simulink model "Six_DoF_LQR"  (R2020b)
settings: Solver=VariableStepAuto  StartTime=0.0  StopTime=6  RelTol=1e-3
values from neighbouring files (symbols this model uses):
  D = zeros(3,2)    [ss_3DoF_LQR.m]    (also in ss_6DoF_LQR.m = zeros(6,2))
  inertiaxx = 0.0015    [Data_for_simulation.m]
  inertiayy = 0.048    [Data_for_simulation.m]
  inertiazz = 0.048    [Data_for_simulation.m]
  K = lqr(A,B,Q,R)    [ss_3DoF_LQR.m]    (also in ss_6DoF_LQR.m)
  mass = 0.8426    [Data_for_simulation.m]
  moment_arm = 0.29    [Data_for_simulation.m]
  tvc_misang = 0    [Data_for_simulation.m]
libraries: simulink_extras x3, shared6dof x1, aerolibutil x1, sharedutil x1
settings Model: Creator=tushark  LastModifiedBy=tushark

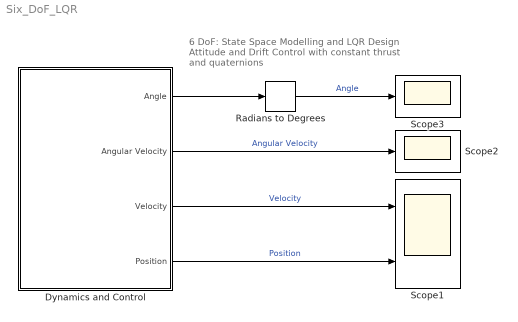
== system Six_DoF_LQR ==
  note: 6 DoF: State Space Modelling and LQR Design
      | Attitude and Drift Control with constant thrust and quaternions
  Dynamics and Control : Subsystem
  Radians to Degrees : simulink_extras/Transformations/Radians to Degrees
  Scope1 : Scope  NumInputPorts=2
  Scope2 : Scope
  Scope3 : Scope
  wires:
  Dynamics and Control/1(Angle) -> Radians to Degrees/1
  Dynamics and Control/2(Angular Velocity) -> Scope2/1  "Angular Velocity"
  Dynamics and Control/3(Velocity) -> Scope1/1  "Velocity"
  Radians to Degrees/1 -> Scope3/1  "Angle"
  Dynamics and Control/4(Position) -> Scope1/2  "Position"

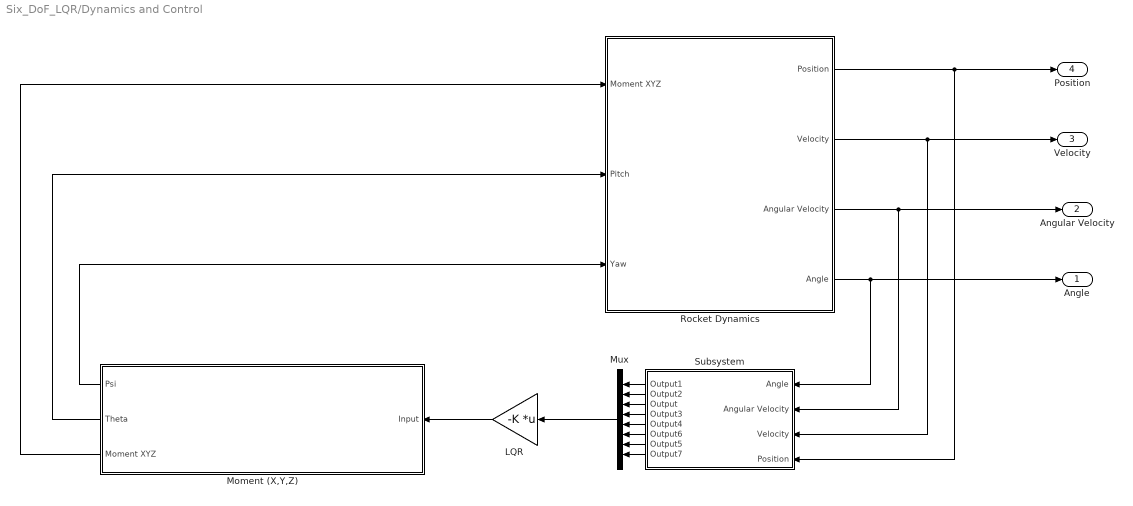
== system Six_DoF_LQR/Dynamics and Control ==
  LQR : Gain  Gain=-K  Multiplication=Matrix(K*u)
  Moment (X,Y,Z) : Subsystem
  Mux : Mux  Inputs=8
  Rocket Dynamics : Subsystem
  Subsystem : Subsystem
  Angle : Outport
  Angular Velocity : Outport  Port=2
  Velocity : Outport  Port=3
  Position : Outport  Port=4
  wires:
  Rocket Dynamics/3(Angular Velocity) -> Angular Velocity/1, Subsystem/2(Angular Velocity)
  Rocket Dynamics/2(Velocity) -> Subsystem/3(Velocity), Velocity/1
  Mux/1 -> LQR/1
  LQR/1 -> Moment (X,Y,Z)/1("Input ")
  Moment (X,Y,Z)/1(Psi) -> Rocket Dynamics/3(Yaw)
  Moment (X,Y,Z)/2(Theta) -> Rocket Dynamics/2(Pitch)
  Moment (X,Y,Z)/3(Moment XYZ) -> Rocket Dynamics/1(Moment XYZ)
  Rocket Dynamics/1(Position) -> Subsystem/4(Position), Position/1
  Rocket Dynamics/4(Angle) -> Subsystem/1(Angle), Angle/1
  Subsystem/1(Output1) -> Mux/1
  Subsystem/2(Output2) -> Mux/2
  Subsystem/3(Output) -> Mux/3
  Subsystem/4(Output3) -> Mux/4
  Subsystem/5(Output4) -> Mux/5
  Subsystem/6(Output6) -> Mux/6
  Subsystem/7(Output5) -> Mux/7
  Subsystem/8(Output7) -> Mux/8

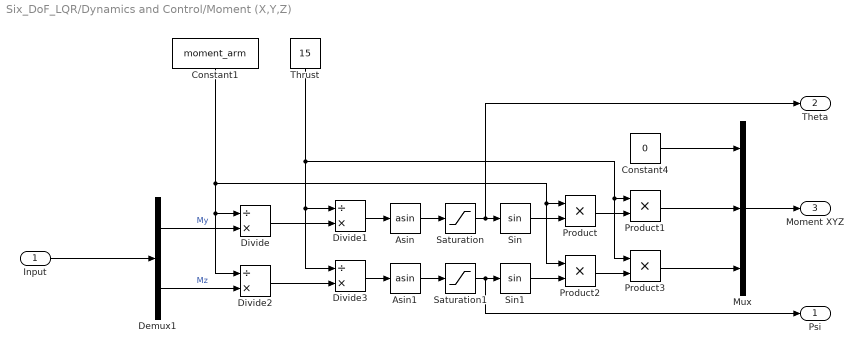
== system Six_DoF_LQR/Dynamics and Control/Moment (X,Y,Z) ==
  "Input " : Inport
  Asin : Trigonometry  Operator=asin
  Asin1 : Trigonometry  Operator=asin
  Constant1 : Constant  Value=moment_arm
  Constant4 : Constant  Value=0
  Demux1 : Demux  Outputs=2
  Divide{,1..3} (4 alike) : Product  Inputs=/*
  Mux : Mux  Inputs=3
  Product{,1..3} (4 alike) : Product
  Saturation : Saturate  UpperLimit=0.174  LowerLimit=-0.174
  Saturation1 : Saturate  UpperLimit=0.174  LowerLimit=-0.174
  Sin : Trigonometry
  Sin1 : Trigonometry
  Thrust : Constant  Value=15
  Psi : Outport
  Theta : Outport  Port=2
  Moment XYZ : Outport  Port=3
  wires:
  Divide/1 -> Divide1/2
  Demux1/1 -> Divide/2  "My"
  Divide1/1 -> Asin/1
  Asin/1 -> Saturation/1
  Saturation/1 -> Theta/1, Sin/1
  Sin/1 -> Product/2
  Product/1 -> Product1/2
  Product1/1 -> Mux/2
  Divide3/1 -> Asin1/1
  Thrust/1 -> Product3/1, Product1/1, Divide1/1, Divide3/1
  Divide2/1 -> Divide3/2
  Constant1/1 -> Product2/1, Product/1, Divide2/1, Divide/1
  Product2/1 -> Product3/2
  Asin1/1 -> Saturation1/1
  Sin1/1 -> Product2/2
  Saturation1/1 -> Psi/1, Sin1/1
  Product3/1 -> Mux/3
  Constant4/1 -> Mux/1
  Mux/1 -> Moment XYZ/1
  Demux1/2 -> Divide2/2  "Mz"
  "Input "/1 -> Demux1/1

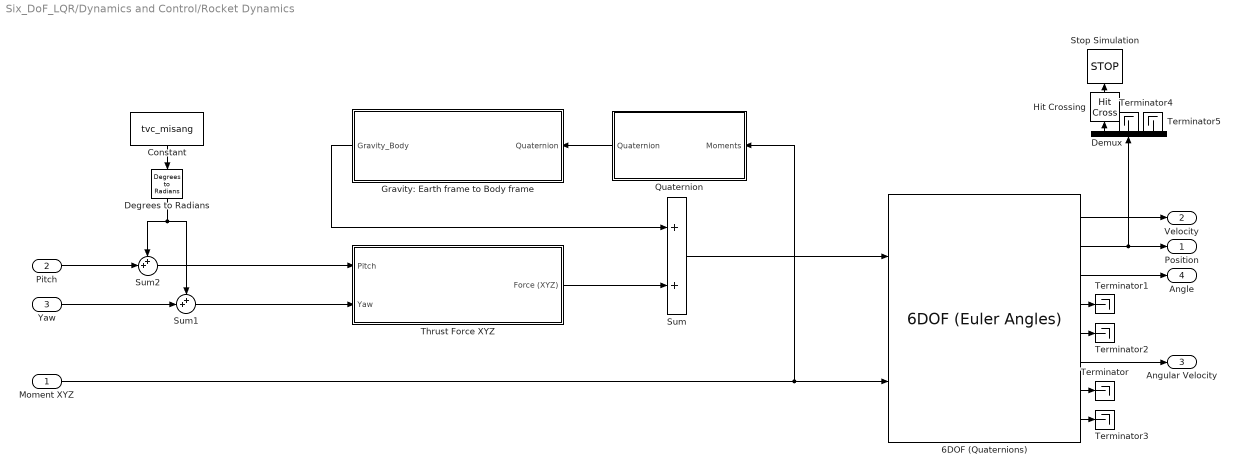
== system Six_DoF_LQR/Dynamics and Control/Rocket Dynamics ==
  Moment XYZ : Inport
  Pitch : Inport  Port=2
  Yaw : Inport  Port=3
  6DOF (Quaternions) : shared6dof/6DOF (Euler Angles)  units=Metric (MKS)  mtype=Fixed  rep=Quaternion  xme_0=[150 0 0]  Vm_0=[0 0 0]  eul_0=[0 0 0]  pm_0=[0 0 0]  mass_0=mass  mass_e=0.5  mass_f=2.0  inertia=[inertiaxx inertiayy inertiazz].*eye(3)  inertia_e=eye(3)  inertia_f=2*eye(3)  k_quat=1.0  vre_flag=on  abi_flag=off  aMode=0  xme_statename=''  Vm_statename=''  eul_statename=''  quat_statename=''  pm_statename=''  mass_statename=''
      settings: SourceProductBaseCode=AE,PW,MT,UV,VE,VP
  Constant : Constant  Value=tvc_misang
  Degrees to Radians : simulink_extras/Transformations/Degrees to Radians
  Demux : Demux  Outputs=3
  Gravity: Earth frame to Body frame : Subsystem
  Hit Crossing : HitCross  HitCrossingDirection=falling
  Quaternion : Subsystem
  Stop Simulation : Stop
  Sum : Sum
  Sum1 : Sum  Inputs=++|
  Sum2 : Sum  Inputs=++|
  Terminator{,1..5} (6 alike) : Terminator
  Thrust Force XYZ : Subsystem
  Position : Outport
  Velocity : Outport  Port=2
  Angular Velocity : Outport  Port=3
  Angle : Outport  Port=4
  wires:
  6DOF (Quaternions)/1 -> Velocity/1
  6DOF (Quaternions)/7 -> Terminator/1
  6DOF (Quaternions)/6 -> Angular Velocity/1
  Sum/1 -> 6DOF (Quaternions)/1
  6DOF (Quaternions)/5 -> Terminator2/1
  Gravity: Earth frame to Body frame/1(Gravity_Body) -> Sum/1
  Thrust Force XYZ/1(Force (XYZ)) -> Sum/2
  6DOF (Quaternions)/8 -> Terminator3/1
  Constant/1 -> Degrees to Radians/1
  Sum1/1 -> Thrust Force XYZ/2(Yaw)
  Sum2/1 -> Thrust Force XYZ/1(Pitch)
  Pitch/1 -> Sum2/2
  Yaw/1 -> Sum1/2
  Degrees to Radians/1 -> Sum2/1, Sum1/1
  6DOF (Quaternions)/3 -> Angle/1
  Quaternion/1(Quaternion) -> Gravity: Earth frame to Body frame/1(Quaternion)
  6DOF (Quaternions)/4 -> Terminator1/1
  Moment XYZ/1 -> Quaternion/1(Moments), 6DOF (Quaternions)/2
  Demux/1 -> Hit Crossing/1
  Demux/2 -> Terminator4/1
  6DOF (Quaternions)/2 -> Demux/1, Position/1
  Hit Crossing/1 -> Stop Simulation/1
  Demux/3 -> Terminator5/1

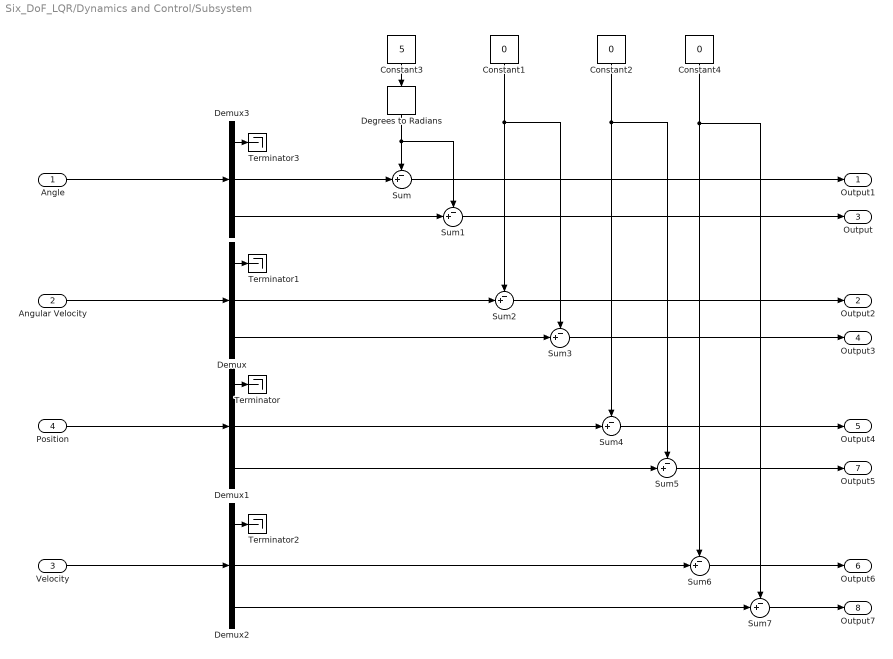
== system Six_DoF_LQR/Dynamics and Control/Subsystem ==
  Angle : Inport
  Angular Velocity : Inport  Port=2
  Velocity : Inport  Port=3
  Position : Inport  Port=4
  Constant1 : Constant  Value=0
  Constant2 : Constant  Value=0
  Constant3 : Constant  Value=5
  Constant4 : Constant  Value=0
  Degrees to Radians : simulink_extras/Transformations/Degrees to Radians
  Demux{,1..3} (4 alike) : Demux  Outputs=3
  Sum{,1..7} (8 alike) : Sum  Inputs=-+|
  Terminator{,1..3} (4 alike) : Terminator
  Output1 : Outport
  Output2 : Outport  Port=2
  Output : Outport  Port=3
  Output3 : Outport  Port=4
  Output4 : Outport  Port=5
  Output6 : Outport  Port=6
  Output5 : Outport  Port=7
  Output7 : Outport  Port=8
  wires:
  Demux/2 -> Sum2/2
  Demux/3 -> Sum3/2
  Demux1/2 -> Sum4/2
  Demux1/3 -> Sum5/2
  Demux1/1 -> Terminator/1
  Demux/1 -> Terminator1/1
  Sum/1 -> Output1/1
  Sum1/1 -> Output/1
  Sum2/1 -> Output2/1
  Sum3/1 -> Output3/1
  Sum4/1 -> Output4/1
  Sum5/1 -> Output5/1
  Angular Velocity/1 -> Demux/1
  Constant1/1 -> Sum3/1, Sum2/1
  Constant2/1 -> Sum5/1, Sum4/1
  Demux2/2 -> Sum6/2
  Demux2/1 -> Terminator2/1
  Sum6/1 -> Output6/1
  Sum7/1 -> Output7/1
  Demux2/3 -> Sum7/2
  Constant4/1 -> Sum7/1, Sum6/1
  Angle/1 -> Demux3/1
  Demux3/2 -> Sum/2
  Demux3/3 -> Sum1/2
  Demux3/1 -> Terminator3/1
  Velocity/1 -> Demux2/1
  Position/1 -> Demux1/1
  Constant3/1 -> Degrees to Radians/1
  Degrees to Radians/1 -> Sum1/1, Sum/1

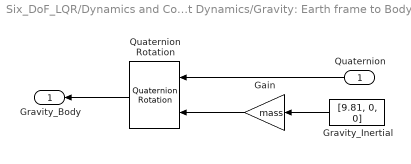
== system Six_DoF_LQR/Dynamics and Control/Rocket Dynamics/Gravity: Earth frame to Body frame ==
  Quaternion : Inport
  Gain : Gain  Gain=mass
  Gravity_Inertial : Constant  Value=[9.81, 0, 0]
  Quaternion Rotation : aerolibutil/Quaternion Rotation
  Gravity_Body : Outport
  wires:
  Gravity_Inertial/1 -> Gain/1
  Gain/1 -> Quaternion Rotation/2
  Quaternion/1 -> Quaternion Rotation/1
  Quaternion Rotation/1 -> Gravity_Body/1

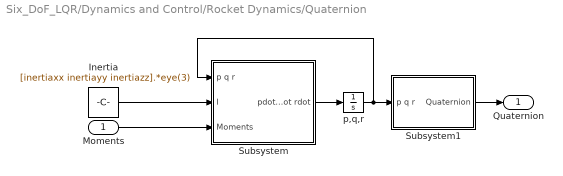
== system Six_DoF_LQR/Dynamics and Control/Rocket Dynamics/Quaternion ==
  Moments : Inport  Unit=N*m  PortDimensions=3
  Inertia : Constant  Value=[inertiaxx inertiayy inertiazz].*eye(3)
  Subsystem : Subsystem
  Subsystem1 : Subsystem
  p,q,r : Integrator
  Quaternion : Outport  VectorParamsAs1DForOutWhenUnconnected=off
  wires:
  p,q,r/1 -> Subsystem1/1(p q r), Subsystem/1(p q r)
  Subsystem1/1(Quaternion) -> Quaternion/1
  Moments/1 -> Subsystem/3(Moments)
  Inertia/1 -> Subsystem/2(I)
  Subsystem/1(pdot qdot rdot) -> p,q,r/1

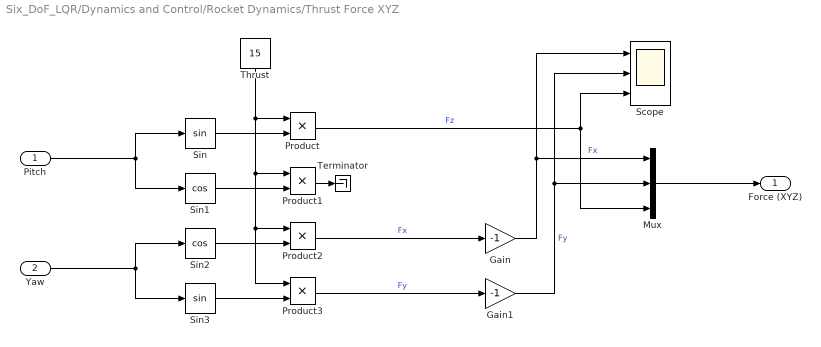
== system Six_DoF_LQR/Dynamics and Control/Rocket Dynamics/Thrust Force XYZ ==
  Pitch : Inport
  Yaw : Inport  Port=2
  Gain : Gain  Gain=-1
  Gain1 : Gain  Gain=-1
  Mux : Mux  Inputs=3
  Product{,1..3} (4 alike) : Product
  Scope : Scope  NumInputPorts=3
  Sin : Trigonometry
  Sin1 : Trigonometry  Operator=cos
  Sin2 : Trigonometry  Operator=cos
  Sin3 : Trigonometry
  Terminator : Terminator
  Thrust : Constant  Value=15
  Force (XYZ) : Outport
  wires:
  Sin2/1 -> Product2/2
  Sin/1 -> Product/2
  Sin1/1 -> Product1/2
  Product3/1 -> Gain1/1  "Fy"
  Product/1 -> Mux/3, Scope/3  "Fz"
  Thrust/1 -> Product/1, Product1/1, Product2/1, Product3/1
  Mux/1 -> Force (XYZ)/1
  Sin3/1 -> Product3/2
  Product2/1 -> Gain/1  "Fx"
  Gain/1 -> Mux/1, Scope/1  "Fx"
  Yaw/1 -> Sin3/1, Sin2/1
  Pitch/1 -> Sin/1, Sin1/1
  Gain1/1 -> Mux/2, Scope/2  "Fy"
  Product1/1 -> Terminator/1

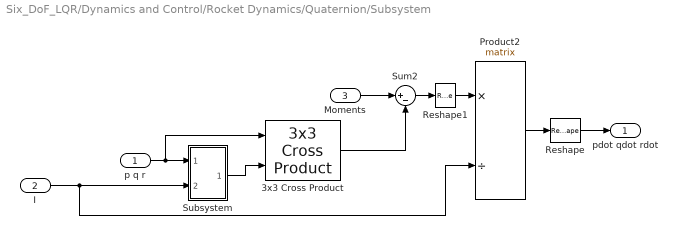
== system Six_DoF_LQR/Dynamics and Control/Rocket Dynamics/Quaternion/Subsystem ==
  p q r : Inport
  I : Inport  Port=2
  Moments : Inport  Port=3
  3x3 Cross Product : sharedutil/3x3 Cross Product  aMode=aMode
      settings: SourceProductBaseCode=AE,PW,MT,UV,VE,VP
  Product2 : Product  Inputs=*/  Multiplication=Matrix(*)  SaturateOnIntegerOverflow=on  OutDataTypeStr=Inherit: Same as first input
  Reshape : Reshape
  Reshape1 : Reshape  OutputDimensionality=Row vector (2-D)
  Subsystem : Subsystem
  Sum2 : Sum  Inputs=|+-  SaturateOnIntegerOverflow=on
  pdot qdot rdot : Outport  VectorParamsAs1DForOutWhenUnconnected=off
  wires:
  Moments/1 -> Sum2/1
  Reshape1/1 -> Product2/1
  I/1 -> Subsystem/2(Inertia), Product2/2
  Sum2/1 -> Reshape1/1
  p q r/1 -> Subsystem/1(p q r1), 3x3 Cross Product/1
  Product2/1 -> Reshape/1
  Reshape/1 -> pdot qdot rdot/1
  Subsystem/1(I * w) -> 3x3 Cross Product/2
  3x3 Cross Product/1 -> Sum2/2

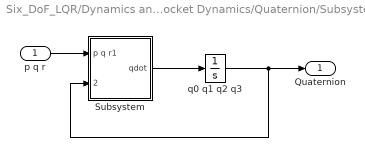
== system Six_DoF_LQR/Dynamics and Control/Rocket Dynamics/Quaternion/Subsystem1 ==
  p q r : Inport
  Subsystem : Subsystem
  q0 q1 q2 q3 : Integrator  InitialCondition=[1, 0, 0, 0]
  Quaternion : Outport  VectorParamsAs1DForOutWhenUnconnected=off
  wires:
  Subsystem/1(qdot) -> q0 q1 q2 q3/1
  p q r/1 -> Subsystem/1(p q r1)
  q0 q1 q2 q3/1 -> Subsystem/2(q0 q1 q2 q3), Quaternion/1

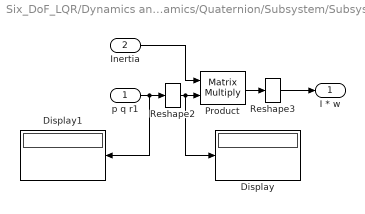
== system Six_DoF_LQR/Dynamics and Control/Rocket Dynamics/Quaternion/Subsystem/Subsystem ==
  p q r1 : Inport
  Inertia : Inport  Port=2
  Display : Display
  Display1 : Display
  Product : Product  Multiplication=Matrix(*)  InputSameDT=on  SaturateOnIntegerOverflow=on  OutDataTypeStr=Inherit: Same as first input
  Reshape2 : Reshape  OutputDimensionality=Column vector (2-D)
  Reshape3 : Reshape
  I * w : Outport  VectorParamsAs1DForOutWhenUnconnected=off
  wires:
  p q r1/1 -> Display1/1, Reshape2/1
  Product/1 -> Reshape3/1
  Inertia/1 -> Product/1
  Reshape2/1 -> Display/1, Product/2
  Reshape3/1 -> I * w/1

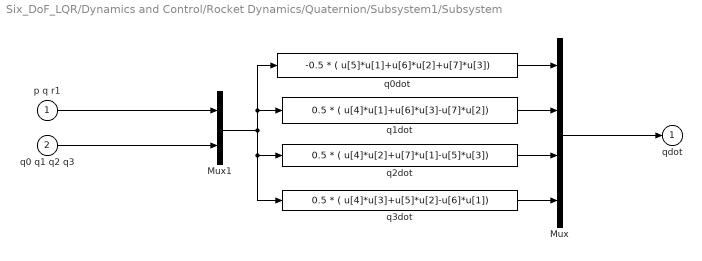
== system Six_DoF_LQR/Dynamics and Control/Rocket Dynamics/Quaternion/Subsystem1/Subsystem ==
  p q r1 : Inport
  q0 q1 q2 q3 : Inport  Port=2  PortDimensions=4
  Mux : Mux
  Mux1 : Mux  Inputs=[3 4]
  q0dot : Fcn  Expr=-0.5 * ( u[5]*u[1]+u[6]*u[2]+u[7]*u[3])
  q1dot : Fcn  Expr=0.5 * ( u[4]*u[1]+u[6]*u[3]-u[7]*u[2])
  q2dot : Fcn  Expr=0.5 * ( u[4]*u[2]+u[7]*u[1]-u[5]*u[3])
  q3dot : Fcn  Expr=0.5 * ( u[4]*u[3]+u[5]*u[2]-u[6]*u[1])
  qdot : Outport  InitialOutput=0  VectorParamsAs1DForOutWhenUnconnected=off
  wires:
  Mux/1 -> qdot/1
  Mux1/1 -> q0dot/1, q1dot/1, q3dot/1, q2dot/1
  p q r1/1 -> Mux1/1
  q0 q1 q2 q3/1 -> Mux1/2
  q0dot/1 -> Mux/1
  q1dot/1 -> Mux/2
  q2dot/1 -> Mux/3
  q3dot/1 -> Mux/4
